simulink model "HVDC_VSC_1CPUcore_dcpl"  (Simulink 8.4)
settings: Solver=ode3  SolverMode=SingleTasking  StartTime=0.0  StopTime=70.0  FixedStep=Ts_Power  RelTol=1e-3  AbsTol=1e-2
PreLoadFcn:
  | Ts_Power=50e-6; Ts_Control=1*Ts_Power; init_cosim_IA; startup_transients_hvdc_vsc;
PostLoadFcn:
  | Ts_Power=50e-6; Ts_Control=1*Ts_Power; init_cosim_IA; startup_transients_hvdc_vsc;
InitFcn:
  | Ts_Power=50e-6; Ts_Control=1*Ts_Power; init_cosim_IA; startup_transients_hvdc_vsc;
values from neighbouring files (symbols this model uses):
  h = 5    [init_cosim_IA.m]
  intfDelay = 400.0    (= 400)    [init_cosim_IA.m]
  Ts_intf = 2*Ts_Power    [init_cosim_IA.m]
undefined symbols (not defined in the file or in its folder): CLARK, D1, Delta, dPref1_2, dPref1_2_rlimit, gcbh, level, lib_mesures, magnitude, ResistanceM, rte_drive_private_lib, rte_tsb3level_hiz_rect_cb, sps_rtmsupport, t_deblock_Pref1, t_deblock_Udref2, t_dPref1_2, t_init_AC, t_SwitchITMIdc, t_SwitchITMVdc, t_vsag_end, t_vsag_start, TSB3_hiZR
libraries: powerlib x162, powerlib_extras x71, spsVIMeasurementModel x63, rteventslib x26, op_dpl_lib x14, powerlib_meascontrol x14, rtlab x6, sps_avr x3, artemis x1
(part 9 of 11)

== system HVDC_VSC_1CPUcore_dcpl/SM_HVDC_VSC/VSC Controller (Station 1)/Discrete VSC Controller (Station 1)/Outer Active-Reactive Power and Voltage Loop/Reactive_Power_Control/AC Voltage Control Override ==
  note: Reset states when enabling
  note: AC Voltage Control Override
  note: Output is added to the regulator reference in order to maintain the AC voltage within minimum and maximum limits
  Ki_rpc_vco : Inport
  Kp_rpc_vco : Inport  Port=2
  U_max : Inport  Port=3
  U_min : Inport  Port=4
  U_meas : Inport  Port=5
  Enable : EnablePort  StatesWhenEnabling=reset
  Constant2 : Constant  Value=0.0
  Constant3 : Constant  Value=min_rpc_vco
  Constant5 : Constant
  Constant6 : Constant  Value=max_rpc_vco
  Constant7 : Constant  Value=0.0
  Constant8 : Constant
  "Int1 " : Subsystem  mask(Integrator  With  External  Dynamic  Limits (Discrete)){i_ic=0, Ts=Ts_Control}
      mask prompts: i_ic "Initial Condition:"; Ts "Sample time: (s)"
      mask Display: disp('Discrete-Time\n(Trapezoidal)\nIntegrator\n ')
  Int2 : Subsystem  mask(Integrator  With  External  Dynamic  Limits (Discrete)){i_ic=0, Ts=Ts_Control}
      mask prompts: i_ic "Initial Condition:"; Ts "Sample time: (s)"
      mask Display: disp('Discrete-Time\n(Trapezoidal)\nIntegrator\n ')
  Logical Operator : Logic  Operator=NOT  Inputs=1  AllPortsSameDT=off
  Logical Operator1 : Logic  Operator=NOT  Inputs=1  AllPortsSameDT=off
  Max=0 Min=min_rpc_vco : Saturate  UpperLimit=0  LowerLimit=min_rpc_vco
  Max=max_rpc_vco Min=0 : Saturate  UpperLimit=max_rpc_vco  LowerLimit=0
  Max=max_rpc_vco Min=min_rpc_vco : Saturate  UpperLimit=max_rpc_vco  LowerLimit=min_rpc_vco
  Product : Product  RndMeth=Zero
  Sum : Sum  Inputs=+-  SaturateOnIntegerOverflow=on
  Sum1 : Sum  Inputs=-+  SaturateOnIntegerOverflow=on
  Sum2 : Sum  Inputs=+++  SaturateOnIntegerOverflow=on
  Sum3 : Sum  SaturateOnIntegerOverflow=on
  Out : Outport
  wires:
  Product/1 -> Sum2/3
  Sum3/1 -> Product/2
  Kp_rpc_vco/1 -> Product/1
  Max=max_rpc_vco Min=0/1 -> Sum3/2
  Int2/1(Out) -> Sum2/2  "positive"
  Max=0 Min=min_rpc_vco/1 -> Sum3/1
  Logical Operator/1 -> "Int1 "/5(Hold), "Int1 "/6(Reset)
  Constant5/1 -> Logical Operator/1
  Constant2/1 -> "Int1 "/1(Max), "Int1 "/7(Reset Value)
  Constant3/1 -> "Int1 "/2(Min)
  Ki_rpc_vco/1 -> Int2/4(Ki), "Int1 "/4(Ki)
  U_max/1 -> Sum/1
  U_meas/1 -> Sum/2, Sum1/1
  Sum/1 -> Max=0 Min=min_rpc_vco/1, "Int1 "/3(In)
  Logical Operator1/1 -> Int2/5(Hold), Int2/6(Reset)
  Constant8/1 -> Logical Operator1/1
  Constant6/1 -> Int2/1(Max)
  Constant7/1 -> Int2/2(Min), Int2/7(Reset Value)
  Sum1/1 -> Max=max_rpc_vco Min=0/1, Int2/3(In)
  U_min/1 -> Sum1/2
  "Int1 "/1(Out) -> Sum2/1  "negative"
  Sum2/1 -> Max=max_rpc_vco Min=min_rpc_vco/1
  Max=max_rpc_vco Min=min_rpc_vco/1 -> Out/1

== system HVDC_VSC_1CPUcore_dcpl/SM_HVDC_VSC/VSC Controller (Station 1)/Discrete VSC Controller (Station 1)/Outer Active-Reactive Power and Voltage Loop/Reactive_Power_Control/Freeze_integrator ==
  note: Freeze Integrator
  note: Low AC voltage level
  U_meas : Inport
  Constant8 : Constant  Value=V_level_rpc
  Relational Operator : RelationalOperator  Operator=<=
  Freeze : Outport
  wires:
  U_meas/1 -> Relational Operator/1
  Relational Operator/1 -> Freeze/1
  Constant8/1 -> Relational Operator/2

== system HVDC_VSC_1CPUcore_dcpl/SM_HVDC_VSC/VSC Controller (Station 1)/Discrete VSC Controller (Station 1)/Outer Active-Reactive Power and Voltage Loop/Reactive_Power_Control/Regulator ==
  note: Regulator
  note: Reset states when enabling
  Ord : Inport
  Meas : Inport  Port=2
  Ki : Inport  Port=3
  max_out : Inport  Port=4
  min_out : Inport  Port=5
  freeze : Inport  Port=6
  Enable : EnablePort  StatesWhenEnabling=reset
  Constant1 : Constant  Value=0
  Constant2 : Constant  Value=max_i_rpc
  Constant3 : Constant  Value=min_i_rpc
  Constant5 : Constant
  Constant7 : Constant  Value=0.0
  Gain : Gain  Gain=-1  SaturateOnIntegerOverflow=on  OutDataTypeStr=Inherit: Same as input  ParamDataTypeStr=Inherit: Same as input
  Ic=0 : UnitDelay  SampleTime=Ts_Control
  Int : Subsystem  mask(Integrator  With  External  Dynamic  Limits (Discrete)){i_ic=0, Ts=Ts_Control}
      mask prompts: i_ic "Initial Condition:"; Ts "Sample time: (s)"
      mask Display: disp('Discrete-Time\n(Trapezoidal)\nIntegrator\n ')
  Kf_rpc : Constant  Value=1.0
  Logical Operator : Logic  Operator=NOT  Inputs=1  AllPortsSameDT=off
  Product2 : Product  SaturateOnIntegerOverflow=on  OutDataTypeStr=Inherit: Same as first input
  S6 : Subsystem  AncestorBlock=|  mask(Limiter with External Limits){}
      | powerlib_extras/Discrete 
      | Control Blocks/Discrete 12-Pulse
      | HVDC Control /Functions
      | (Discrete)/Current Regulator/S16/S6
      mask Display: disp('      Limiter\n')
  Sum1 : Sum  SaturateOnIntegerOverflow=on
  Sum2 : Sum  Inputs=|+-  SaturateOnIntegerOverflow=on
  Sum3 : Sum  SaturateOnIntegerOverflow=on
  Sum4 : Sum  Inputs=+-  SaturateOnIntegerOverflow=on
  Switch : Switch  Threshold=0.5  SaturateOnIntegerOverflow=on
  Out : Outport
  wires:
  Gain/1 -> Out/1
  Ic=0/1 -> Sum1/2
  Kf_rpc/1 -> Product2/1
  Logical Operator/1 -> Int/5(Hold), Int/6(Reset)
  Constant5/1 -> Logical Operator/1
  Constant1/1 -> Int/7(Reset Value)
  Constant2/1 -> Int/1(Max)
  Constant3/1 -> Int/2(Min)
  Sum1/1 -> Int/3(In)
  Ord/1 -> Sum3/1, Sum4/1
  Ki/1 -> Int/4(Ki)
  max_out/1 -> S6/1(MAX)
  min_out/1 -> S6/3(MIN)
  S6/1("  ") -> Gain/1, Sum2/1
  Sum2/1 -> Product2/2
  Product2/1 -> Ic=0/1
  Sum3/1 -> S6/2(In), Sum2/2
  Int/1(Out) -> Sum3/2
  freeze/1 -> Switch/2
  Constant7/1 -> Switch/1
  Sum4/1 -> Switch/3
  Switch/1 -> Sum1/1
  Meas/1 -> Sum4/2

== system HVDC_VSC_1CPUcore_dcpl/SM_HVDC_VSC/VSC Controller (Station 2)/Discrete VSC Controller (Station 2)/Clark Transformations/CLARK_YD/CLARK ==
  note: CLARK transformation
  abc : Inport
  Enable : EnablePort
  Fcn1 : Fcn  Expr=1/sqrt(3)*(u[2] - u[3])
  Fcn2 : Fcn  Expr=1/3*(2*u[1] - u[2] - u[3])
  Fcn3 : Fcn  Expr=1/3*(u[1] + u[2] + u[3])
  Mux : Mux  Inputs=3
  AB0 : Outport
  wires:
  Fcn2/1 -> Mux/1
  abc/1 -> Fcn1/1, Fcn3/1, Fcn2/1
  Fcn1/1 -> Mux/2
  Fcn3/1 -> Mux/3
  Mux/1 -> AB0/1

== system HVDC_VSC_1CPUcore_dcpl/SM_HVDC_VSC/VSC Controller (Station 2)/Discrete VSC Controller (Station 2)/Clark Transformations/CLARK_YD/CLARK_YD1 ==
  note: CLARK transformation - YD1
  abc : Inport
  Enable : EnablePort
  Fcn1 : Fcn  Expr=(-u[1] - u[3] + 2*u[2] )/3
  Fcn2 : Fcn  Expr=(u[1]-u[3])/sqrt(3)
  Fcn3 : Fcn  Expr=0
  Mux : Mux  Inputs=3
  AB0 : Outport
  wires:
  Fcn2/1 -> Mux/1
  abc/1 -> Fcn1/1, Fcn3/1, Fcn2/1
  Fcn1/1 -> Mux/2
  Fcn3/1 -> Mux/3
  Mux/1 -> AB0/1

== system HVDC_VSC_1CPUcore_dcpl/SM_HVDC_VSC/VSC Controller (Station 2)/Discrete VSC Controller (Station 2)/Clark Transformations/CLARK_YD/CLARK_YD11 ==
  note: CLARK transformation - YD11
  abc : Inport
  Enable : EnablePort
  Fcn1 : Fcn  Expr=(u[1] + u[2] - 2*u[3] )/3
  Fcn2 : Fcn  Expr=(u[1]-u[2])/sqrt(3)
  Fcn3 : Fcn  Expr=0
  Mux : Mux  Inputs=3
  AB0 : Outport
  wires:
  Mux/1 -> AB0/1
  Fcn3/1 -> Mux/3
  Fcn1/1 -> Mux/2
  abc/1 -> Fcn2/1, Fcn3/1, Fcn1/1
  Fcn2/1 -> Mux/1

== system HVDC_VSC_1CPUcore_dcpl/SM_HVDC_VSC/VSC Controller (Station 2)/Discrete VSC Controller (Station 2)/Clark Transformations/CLARK_YD /CLARK ==
  note: CLARK transformation
  abc : Inport
  Enable : EnablePort
  Fcn1 : Fcn  Expr=1/sqrt(3)*(u[2] - u[3])
  Fcn2 : Fcn  Expr=1/3*(2*u[1] - u[2] - u[3])
  Fcn3 : Fcn  Expr=1/3*(u[1] + u[2] + u[3])
  Mux : Mux  Inputs=3
  AB0 : Outport
  wires:
  Mux/1 -> AB0/1
  Fcn3/1 -> Mux/3
  Fcn1/1 -> Mux/2
  abc/1 -> Fcn2/1, Fcn3/1, Fcn1/1
  Fcn2/1 -> Mux/1

== system HVDC_VSC_1CPUcore_dcpl/SM_HVDC_VSC/VSC Controller (Station 2)/Discrete VSC Controller (Station 2)/Clark Transformations/CLARK_YD /CLARK_YD1 ==
  note: CLARK transformation - YD1
  abc : Inport
  Enable : EnablePort
  Fcn1 : Fcn  Expr=(-u[1] - u[3] + 2*u[2] )/3
  Fcn2 : Fcn  Expr=(u[1]-u[3])/sqrt(3)
  Fcn3 : Fcn  Expr=0
  Mux : Mux  Inputs=3
  AB0 : Outport
  wires:
  Mux/1 -> AB0/1
  Fcn3/1 -> Mux/3
  Fcn1/1 -> Mux/2
  abc/1 -> Fcn2/1, Fcn3/1, Fcn1/1
  Fcn2/1 -> Mux/1

== system HVDC_VSC_1CPUcore_dcpl/SM_HVDC_VSC/VSC Controller (Station 2)/Discrete VSC Controller (Station 2)/Clark Transformations/CLARK_YD /CLARK_YD11 ==
  note: CLARK transformation - YD11
  abc : Inport
  Enable : EnablePort
  Fcn1 : Fcn  Expr=(u[1] + u[2] - 2*u[3] )/3
  Fcn2 : Fcn  Expr=(u[1]-u[2])/sqrt(3)
  Fcn3 : Fcn  Expr=0
  Mux : Mux  Inputs=3
  AB0 : Outport
  wires:
  Fcn2/1 -> Mux/1
  abc/1 -> Fcn1/1, Fcn3/1, Fcn2/1
  Fcn1/1 -> Mux/2
  Fcn3/1 -> Mux/3
  Mux/1 -> AB0/1

== system HVDC_VSC_1CPUcore_dcpl/SM_HVDC_VSC/VSC Controller (Station 2)/Discrete VSC Controller (Station 2)/DC Voltage Balance Control/Regulator/PI_regulator  ==
  note: PI Regulator - Type 2
  note: Active Power Control
  note: max_i_apc
  note: min_i_apc
  note: Parameters
  note: Constants
  note: Ki_apc
  note: Kp_apc
  Ord : Inport
  Meas : Inport  Port=2
  Ki : Inport  Port=3
  Kp : Inport  Port=4
  Kf : Inport  Port=5
  Constant1 : Constant  Value=0
  Constant2 : Constant  Value=max_i
  Constant3 : Constant  Value=min_i
  Constant4 : Constant  Value=max_out
  Constant5 : Constant
  Constant6 : Constant  Value=min_out
  INT : Subsystem  mask(Integrator  With  External  Dynamic  Limits (Discrete)){}
      mask Display: disp('Discrete-Time\n(Trapezoidal)\nIntegrator\n ')
  Ic=0 : UnitDelay  SampleTime=Ts
  Logical Operator : Logic  Operator=NOT  Inputs=1  AllPortsSameDT=off
  Product1 : Product  SaturateOnIntegerOverflow=on  OutDataTypeStr=Inherit: Same as first input
  Product2 : Product  SaturateOnIntegerOverflow=on  OutDataTypeStr=Inherit: Same as first input
  S6 : Subsystem  AncestorBlock=|  mask(Limiter with External Limits){}
      | powerlib_extras/Discrete 
      | Control Blocks/Discrete 12-Pulse
      | HVDC Control /Functions
      | (Discrete)/Current Regulator/S16/S6
      mask Display: disp('      Limiter\n')
  Sum2 : Sum  Inputs=|+-  SaturateOnIntegerOverflow=on
  Sum3 : Sum  SaturateOnIntegerOverflow=on
  Sum4 : Sum  Inputs=+-  SaturateOnIntegerOverflow=on
  Sum5 : Sum  SaturateOnIntegerOverflow=on
  Out : Outport
  wires:
  Logical Operator/1 -> INT/6(Reset), INT/5(Hold)
  Constant5/1 -> Logical Operator/1
  Constant1/1 -> INT/7(Reset Value)
  Constant2/1 -> INT/1(Max)
  Constant3/1 -> INT/2(Min)
  Sum4/1 -> Product1/2, Sum5/1
  Meas/1 -> Sum4/2
  Ord/1 -> Sum4/1
  Ki/1 -> INT/4(Ki)
  Constant4/1 -> S6/1(MAX)
  Constant6/1 -> S6/3(MIN)
  S6/1("  ") -> Sum2/1, Out/1
  Sum2/1 -> Product2/2
  Product2/1 -> Ic=0/1
  Kf/1 -> Product2/1
  Ic=0/1 -> Sum5/2
  Sum3/1 -> S6/2(In), Sum2/2
  INT/1(Out) -> Sum3/2
  Kp/1 -> Product1/1
  Sum5/1 -> INT/3(In)
  Product1/1 -> Sum3/1

== system HVDC_VSC_1CPUcore_dcpl/SM_HVDC_VSC/VSC Controller (Station 2)/Discrete VSC Controller (Station 2)/Inner Current Loop/AC_Current_Control/PI_regulator  ==
  note: Kp_apc
  note: Ki_apc
  note: Constants
  note: Parameters
  note: min_i_apc
  note: max_i_apc
  note: Active Power Control
  note: PI Regulator - Type 2
  Ord : Inport
  Meas : Inport  Port=2
  Ki : Inport  Port=3
  Kp : Inport  Port=4
  Kf : Inport  Port=5
  Constant1 : Constant  Value=0
  Constant2 : Constant  Value=max_i
  Constant3 : Constant  Value=min_i
  Constant4 : Constant  Value=max_out
  Constant5 : Constant
  Constant6 : Constant  Value=min_out
  INT : Subsystem  mask(Integrator  With  External  Dynamic  Limits (Discrete)){}
      mask Display: disp('Discrete-Time\n(Trapezoidal)\nIntegrator\n ')
  Ic=0 : UnitDelay  SampleTime=Ts
  Logical Operator : Logic  Operator=NOT  Inputs=1  AllPortsSameDT=off
  Product1 : Product  SaturateOnIntegerOverflow=on  OutDataTypeStr=Inherit: Same as first input
  Product2 : Product  SaturateOnIntegerOverflow=on  OutDataTypeStr=Inherit: Same as first input
  S6 : Subsystem  AncestorBlock=|  mask(Limiter with External Limits){}
      | powerlib_extras/Discrete 
      | Control Blocks/Discrete 12-Pulse
      | HVDC Control /Functions
      | (Discrete)/Current Regulator/S16/S6
      mask Display: disp('      Limiter\n')
  Sum2 : Sum  Inputs=|+-  SaturateOnIntegerOverflow=on
  Sum3 : Sum  SaturateOnIntegerOverflow=on
  Sum4 : Sum  Inputs=+-  SaturateOnIntegerOverflow=on
  Sum5 : Sum  SaturateOnIntegerOverflow=on
  Out : Outport
  wires:
  Product1/1 -> Sum3/1
  Sum5/1 -> INT/3(In)
  Kp/1 -> Product1/1
  INT/1(Out) -> Sum3/2
  Sum3/1 -> Sum2/2, S6/2(In)
  Ic=0/1 -> Sum5/2
  Kf/1 -> Product2/1
  Product2/1 -> Ic=0/1
  Sum2/1 -> Product2/2
  S6/1("  ") -> Out/1, Sum2/1
  Constant6/1 -> S6/3(MIN)
  Constant4/1 -> S6/1(MAX)
  Ki/1 -> INT/4(Ki)
  Ord/1 -> Sum4/1
  Meas/1 -> Sum4/2
  Sum4/1 -> Sum5/1, Product1/2
  Constant3/1 -> INT/2(Min)
  Constant2/1 -> INT/1(Max)
  Constant1/1 -> INT/7(Reset Value)
  Constant5/1 -> Logical Operator/1
  Logical Operator/1 -> INT/5(Hold), INT/6(Reset)

== system HVDC_VSC_1CPUcore_dcpl/SM_HVDC_VSC/VSC Controller (Station 2)/Discrete VSC Controller (Station 2)/Inner Current Loop/AC_Current_Control/PI_regulator_2 ==
  note: PI Regulator - Type 2
  note: Active Power Control
  note: max_i_apc
  note: min_i_apc
  note: Parameters
  note: Constants
  note: Ki_apc
  note: Kp_apc
  Ord : Inport
  Meas : Inport  Port=2
  Ki : Inport  Port=3
  Kp : Inport  Port=4
  Kf : Inport  Port=5
  Constant1 : Constant  Value=0
  Constant2 : Constant  Value=max_i
  Constant3 : Constant  Value=min_i
  Constant4 : Constant  Value=max_out
  Constant5 : Constant
  Constant6 : Constant  Value=min_out
  INT : Subsystem  mask(Integrator  With  External  Dynamic  Limits (Discrete)){}
      mask Display: disp('Discrete-Time\n(Trapezoidal)\nIntegrator\n ')
  Ic=0 : UnitDelay  SampleTime=Ts
  Logical Operator : Logic  Operator=NOT  Inputs=1  AllPortsSameDT=off
  Product1 : Product  SaturateOnIntegerOverflow=on  OutDataTypeStr=Inherit: Same as first input
  Product2 : Product  SaturateOnIntegerOverflow=on  OutDataTypeStr=Inherit: Same as first input
  S6 : Subsystem  AncestorBlock=|  mask(Limiter with External Limits){}
      | powerlib_extras/Discrete 
      | Control Blocks/Discrete 12-Pulse
      | HVDC Control /Functions
      | (Discrete)/Current Regulator/S16/S6
      mask Display: disp('      Limiter\n')
  Sum2 : Sum  Inputs=|+-  SaturateOnIntegerOverflow=on
  Sum3 : Sum  SaturateOnIntegerOverflow=on
  Sum4 : Sum  Inputs=+-  SaturateOnIntegerOverflow=on
  Sum5 : Sum  SaturateOnIntegerOverflow=on
  Out : Outport
  wires:
  Logical Operator/1 -> INT/6(Reset), INT/5(Hold)
  Constant5/1 -> Logical Operator/1
  Constant1/1 -> INT/7(Reset Value)
  Constant2/1 -> INT/1(Max)
  Constant3/1 -> INT/2(Min)
  Sum4/1 -> Product1/2, Sum5/1
  Meas/1 -> Sum4/2
  Ord/1 -> Sum4/1
  Ki/1 -> INT/4(Ki)
  Constant4/1 -> S6/1(MAX)
  Constant6/1 -> S6/3(MIN)
  S6/1("  ") -> Sum2/1, Out/1
  Sum2/1 -> Product2/2
  Product2/1 -> Ic=0/1
  Kf/1 -> Product2/1
  Ic=0/1 -> Sum5/2
  Sum3/1 -> S6/2(In), Sum2/2
  INT/1(Out) -> Sum3/2
  Kp/1 -> Product1/1
  Sum5/1 -> INT/3(In)
  Product1/1 -> Sum3/1

== system HVDC_VSC_1CPUcore_dcpl/SM_HVDC_VSC/VSC Controller (Station 2)/Discrete VSC Controller (Station 2)/Outer Active-Reactive Power and Voltage Loop/Active_Power_Control/DC Voltage Control Override ==
  note: Output is added to the regulator reference in order to maintain the DC voltage within minimum and maximum limits
  note: DC Voltage Control Override
  note: Reset states when enabling
  Ki_apc_vco : Inport
  Kp_apc_vco : Inport  Port=2
  Udc_max : Inport  Port=3
  Udc_min : Inport  Port=4
  Udc_meas : Inport  Port=5
  Enable : EnablePort  StatesWhenEnabling=reset
  Constant2 : Constant  Value=0.0
  Constant3 : Constant  Value=min_apc_vco
  Constant5 : Constant
  Constant6 : Constant  Value=max_apc_vco
  Constant7 : Constant  Value=0.0
  Constant8 : Constant
  "Int1 " : Subsystem  mask(Integrator  With  External  Dynamic  Limits (Discrete)){i_ic=0, Ts=Ts_Control}
      mask prompts: i_ic "Initial Condition:"; Ts "Sample time: (s)"
      mask Display: disp('Discrete-Time\n(Trapezoidal)\nIntegrator\n ')
  Int2 : Subsystem  mask(Integrator  With  External  Dynamic  Limits (Discrete)){i_ic=0, Ts=Ts_Control}
      mask prompts: i_ic "Initial Condition:"; Ts "Sample time: (s)"
      mask Display: disp('Discrete-Time\n(Trapezoidal)\nIntegrator\n ')
  Logical Operator : Logic  Operator=NOT  Inputs=1  AllPortsSameDT=off
  Logical Operator1 : Logic  Operator=NOT  Inputs=1  AllPortsSameDT=off
  Max=0 Min=min_apc_vco : Saturate  UpperLimit=0  LowerLimit=min_apc_vco
  Max=max_apc_vco Min=0 : Saturate  UpperLimit=max_apc_vco  LowerLimit=0
  Max=max_apc_vco Min=min_apc_vco : Saturate  UpperLimit=max_apc_vco  LowerLimit=min_apc_vco
  Product : Product  RndMeth=Zero
  Sum : Sum  Inputs=+-  SaturateOnIntegerOverflow=on
  Sum1 : Sum  Inputs=-+  SaturateOnIntegerOverflow=on
  Sum2 : Sum  Inputs=+++  SaturateOnIntegerOverflow=on
  Sum3 : Sum  SaturateOnIntegerOverflow=on
  Out : Outport
  wires:
  Sum2/1 -> Max=max_apc_vco Min=min_apc_vco/1
  "Int1 "/1(Out) -> Sum2/1  "negative"
  Udc_min/1 -> Sum1/2
  Sum1/1 -> Int2/3(In), Max=max_apc_vco Min=0/1
  Constant7/1 -> Int2/7(Reset Value), Int2/2(Min)
  Constant6/1 -> Int2/1(Max)
  Constant8/1 -> Logical Operator1/1
  Logical Operator1/1 -> Int2/6(Reset), Int2/5(Hold)
  Sum/1 -> "Int1 "/3(In), Max=0 Min=min_apc_vco/1
  Udc_meas/1 -> Sum1/1, Sum/2
  Udc_max/1 -> Sum/1
  Ki_apc_vco/1 -> "Int1 "/4(Ki), Int2/4(Ki)
  Constant3/1 -> "Int1 "/2(Min)
  Constant2/1 -> "Int1 "/7(Reset Value), "Int1 "/1(Max)
  Constant5/1 -> Logical Operator/1
  Logical Operator/1 -> "Int1 "/6(Reset), "Int1 "/5(Hold)
  Max=0 Min=min_apc_vco/1 -> Sum3/1
  Int2/1(Out) -> Sum2/2  "positive"
  Max=max_apc_vco Min=0/1 -> Sum3/2
  Kp_apc_vco/1 -> Product/1
  Sum3/1 -> Product/2
  Product/1 -> Sum2/3
  Max=max_apc_vco Min=min_apc_vco/1 -> Out/1

== system HVDC_VSC_1CPUcore_dcpl/SM_HVDC_VSC/VSC Controller (Station 2)/Discrete VSC Controller (Station 2)/Outer Active-Reactive Power and Voltage Loop/Active_Power_Control/Freeze_integrator ==
  note: Low AC voltage level
  note: Freeze Integrator
  U_meas : Inport
  Constant8 : Constant  Value=V_level_apc
  Relational Operator : RelationalOperator  Operator=<=
  Freeze : Outport
  wires:
  Constant8/1 -> Relational Operator/2
  Relational Operator/1 -> Freeze/1
  U_meas/1 -> Relational Operator/1

== system HVDC_VSC_1CPUcore_dcpl/SM_HVDC_VSC/VSC Controller (Station 2)/Discrete VSC Controller (Station 2)/Outer Active-Reactive Power and Voltage Loop/Active_Power_Control/Ramping ==
  note: Output is reset to zero when the ramp is not enabled
  note: Ramping
  enable_ramp : Inport
  Pref : Inport  Port=2
  ramp_apc : Inport  Port=3
  Logical Operator7 : Logic  Operator=NOT  AllPortsSameDT=off
  Rate Limiter : Subsystem  AncestorBlock=my_linear/Rate Limiter (external)  mask(Rate of Change Limiter){ic=0, st=Ts_Control}
      mask prompts: ic "Initial condition (pu):"; st "Sample time (s):"
      mask help: Limit rising and falling rates of signal. When the input (R) is true the output is reset to the input (In). Rates are in p.u./s for up and -p.u./s for down.
      mask Display: disp('                Rate\n               Limiter')
  Switch : Switch  Threshold=0.5  SaturateOnIntegerOverflow=on
  zero : Constant  Value=0.0
  Pref_ramp : Outport
  wires:
  Logical Operator7/1 -> Rate Limiter/4(R)
  Switch/1 -> Rate Limiter/1(In)
  zero/1 -> Switch/3
  Pref/1 -> Switch/1
  enable_ramp/1 -> Logical Operator7/1, Switch/2
  ramp_apc/1 -> Rate Limiter/2(up_rate), Rate Limiter/3(down_rate)
  Rate Limiter/1(" ") -> Pref_ramp/1

== system HVDC_VSC_1CPUcore_dcpl/SM_HVDC_VSC/VSC Controller (Station 2)/Discrete VSC Controller (Station 2)/Outer Active-Reactive Power and Voltage Loop/Active_Power_Control/Regulator ==
  note: Regulator
  note: Reset states when enabling
  Ord : Inport
  Meas : Inport  Port=2
  Ki : Inport  Port=3
  max_out : Inport  Port=4
  min_out : Inport  Port=5
  Freeze : Inport  Port=6
  Enable : EnablePort  StatesWhenEnabling=reset
  Constant1 : Constant  Value=0
  Constant2 : Constant  Value=max_i_apc
  Constant3 : Constant  Value=min_i_apc
  Constant5 : Constant
  Constant9 : Constant  Value=0.0
  Ic=0 : UnitDelay  SampleTime=Ts_Control
  Int : Subsystem  mask(Integrator  With  External  Dynamic  Limits (Discrete)){i_ic=0, Ts=Ts_Control}
      mask prompts: i_ic "Initial Condition:"; Ts "Sample time: (s)"
      mask Display: disp('Discrete-Time\n(Trapezoidal)\nIntegrator\n ')
  Kf_apc : Constant  Value=1.0
  Logical Operator : Logic  Operator=NOT  Inputs=1  AllPortsSameDT=off
  Product2 : Product  SaturateOnIntegerOverflow=on  OutDataTypeStr=Inherit: Same as first input
  S6 : Subsystem  AncestorBlock=|  mask(Limiter with External Limits){}
      | powerlib_extras/Discrete 
      | Control Blocks/Discrete 12-Pulse
      | HVDC Control /Functions
      | (Discrete)/Current Regulator/S16/S6
      mask Display: disp('      Limiter\n')
  Sum1 : Sum  SaturateOnIntegerOverflow=on
  Sum2 : Sum  Inputs=|+-  SaturateOnIntegerOverflow=on
  Sum3 : Sum  SaturateOnIntegerOverflow=on
  Sum4 : Sum  Inputs=+-  SaturateOnIntegerOverflow=on
  Switch : Switch  Threshold=0.5  SaturateOnIntegerOverflow=on
  Out : Outport
  wires:
  Constant9/1 -> Switch/1
  Freeze/1 -> Switch/2
  Switch/1 -> Sum1/1
  Int/1(Out) -> Sum3/2
  Sum3/1 -> S6/2(In), Sum2/2
  Product2/1 -> Ic=0/1
  Sum2/1 -> Product2/2
  S6/1("  ") -> Sum2/1, Out/1
  min_out/1 -> S6/3(MIN)
  max_out/1 -> S6/1(MAX)
  Ki/1 -> Int/4(Ki)
  Sum1/1 -> Int/3(In)
  Constant3/1 -> Int/2(Min)
  Constant2/1 -> Int/1(Max)
  Constant1/1 -> Int/7(Reset Value)
  Constant5/1 -> Logical Operator/1
  Logical Operator/1 -> Int/6(Reset), Int/5(Hold)
  Kf_apc/1 -> Product2/1
  Ic=0/1 -> Sum1/2
  Ord/1 -> Sum4/1, Sum3/1
  Meas/1 -> Sum4/2
  Sum4/1 -> Switch/3

== system HVDC_VSC_1CPUcore_dcpl/SM_HVDC_VSC/VSC Controller (Station 2)/Discrete VSC Controller (Station 2)/Outer Active-Reactive Power and Voltage Loop/Current_Reference_Calculation/S1 ==
  note: Limiter
      | with external
      | limits
  MAX : Inport
  In : Inport  Port=2
  MIN : Inport  Port=3
  MinMax : MinMax  Function=max  Inputs=2  SaturateOnIntegerOverflow=on  InputSameDT=on
  MinMax1 : MinMax  Inputs=2  SaturateOnIntegerOverflow=on  InputSameDT=on
  "  " : Outport  InitialOutput=0
  wires:
  MinMax1/1 -> MinMax/2
  MAX/1 -> MinMax1/1
  MIN/1 -> MinMax/1
  MinMax/1 -> "  "/1
  In/1 -> MinMax1/2

== system HVDC_VSC_1CPUcore_dcpl/SM_HVDC_VSC/VSC Controller (Station 2)/Discrete VSC Controller (Station 2)/Outer Active-Reactive Power and Voltage Loop/Current_Reference_Calculation/S2 ==
  note: Limiter
      | with external
      | limits
  MAX : Inport
  In : Inport  Port=2
  MIN : Inport  Port=3
  MinMax : MinMax  Function=max  Inputs=2  SaturateOnIntegerOverflow=on  InputSameDT=on
  MinMax1 : MinMax  Inputs=2  SaturateOnIntegerOverflow=on  InputSameDT=on
  "  " : Outport  InitialOutput=0
  wires:
  In/1 -> MinMax1/2
  MinMax/1 -> "  "/1
  MIN/1 -> MinMax/1
  MAX/1 -> MinMax1/1
  MinMax1/1 -> MinMax/2

== system HVDC_VSC_1CPUcore_dcpl/SM_HVDC_VSC/VSC Controller (Station 2)/Discrete VSC Controller (Station 2)/Outer Active-Reactive Power and Voltage Loop/Current_Reference_Limitation/Double click here for  info ==
  note: Power System Simulation laboratory (IREQ)
  note: Current Reference Limitation
  note: The susbsytem limits the amplitude of phase current of the fundamental component to the rated current
      | of the converter.
  note: Power Control Mode
  note: DC Voltage Control Mode
  note: In power control mode, equal scaling is applied to the active and reactive power reference when a limit is imposed.
  note: In DC voltage control mode, higher priority is given to the active power when a limit is imposed.

== system HVDC_VSC_1CPUcore_dcpl/SM_HVDC_VSC/VSC Controller (Station 2)/Discrete VSC Controller (Station 2)/Outer Active-Reactive Power and Voltage Loop/DC_Voltage_Control/PI ==
  note: INTEGRATOR (Trapezoidal) with External limits & Reset & Hold
  Max : Inport
  Min : Inport  Port=2
  In : Inport  Port=3
  Ki : Inport  Port=4
  Hold : Inport  Port=5
  Reset : Inport  Port=6
  Reset Value : Inport  Port=7
  Gain : Gain  Gain=Ts* 0.5  SaturateOnIntegerOverflow=on  OutDataTypeStr=Inherit: Same as input  ParamDataTypeStr=Inherit: Same as input
  IC = 0 : UnitDelay  SampleTime=Ts
  IC = i_ic : UnitDelay  InitialCondition=i_ic  SampleTime=Ts
  Logical Operator4 : Logic  Operator=OR
  MinMax : MinMax  Inputs=2  SaturateOnIntegerOverflow=on  InputSameDT=on
  MinMax1 : MinMax  Function=max  Inputs=2  SaturateOnIntegerOverflow=on  InputSameDT=on
  Product : Product  SaturateOnIntegerOverflow=on  OutDataTypeStr=Inherit: Same as first input
  S6 : Subsystem  AncestorBlock=|  mask(Limiter with External Limits){}
      | powerlib_extras/Discrete 
      | Control Blocks/Discrete 12-Pulse
      | HVDC Control /Functions
      | (Discrete)/Current Regulator/S16/S6
      mask Display: disp('      Limiter\n')
  Sum : Sum  SaturateOnIntegerOverflow=on  InputSameDT=on  OutDataTypeStr=Inherit: Same as first input
  Sum1 : Sum  SaturateOnIntegerOverflow=on  InputSameDT=on  OutDataTypeStr=Inherit: Same as first input
  Switch2 : Switch  Threshold=0.5  SaturateOnIntegerOverflow=on  InputSameDT=on
  Switch3 : Switch  Threshold=0.5  SaturateOnIntegerOverflow=on  InputSameDT=on
  Switch7 : Switch  Threshold=0.5  SaturateOnIntegerOverflow=on  InputSameDT=on
  Out : Outport  InitialOutput=0
  wires:
  S6/1("  ") -> IC = i_ic/1, Out/1
  Gain/1 -> Product/1
  Sum1/1 -> Product/2
  Ki/1 -> Gain/1
  IC = 0/1 -> Sum1/2
  In/1 -> IC = 0/1, Sum1/1
  Product/1 -> Sum/1
  Sum/1 -> S6/2(In)
  Hold/1 -> Logical Operator4/1
  Reset/1 -> Switch7/2, Logical Operator4/2
  Logical Operator4/1 -> Switch2/2, Switch3/2
  Switch2/1 -> MinMax/1
  Max/1 -> Switch2/3, MinMax/2
  Reset Value/1 -> Switch7/1
  MinMax/1 -> S6/1(MAX)
  MinMax1/1 -> S6/3(MIN)
  Switch3/1 -> MinMax1/1
  Min/1 -> Switch3/3, MinMax1/2
  IC = i_ic/1 -> Switch7/3
  Switch7/1 -> Switch2/1, Sum/2, Switch3/1

== system HVDC_VSC_1CPUcore_dcpl/SM_HVDC_VSC/VSC Controller (Station 2)/Discrete VSC Controller (Station 2)/Outer Active-Reactive Power and Voltage Loop/DC_Voltage_Control/S6 ==
  note: Limiter
      | with external
      | limits
  MAX : Inport
  In : Inport  Port=2
  MIN : Inport  Port=3
  MinMax : MinMax  Function=max  Inputs=2  SaturateOnIntegerOverflow=on  InputSameDT=on
  MinMax1 : MinMax  Inputs=2  SaturateOnIntegerOverflow=on  InputSameDT=on
  "  " : Outport  InitialOutput=0
  wires:
  MinMax1/1 -> MinMax/2
  MAX/1 -> MinMax1/1
  MIN/1 -> MinMax/1
  MinMax/1 -> "  "/1
  In/1 -> MinMax1/2

== system HVDC_VSC_1CPUcore_dcpl/SM_HVDC_VSC/VSC Controller (Station 2)/Discrete VSC Controller (Station 2)/Outer Active-Reactive Power and Voltage Loop/Reactive_Power_Control/AC Voltage Control Override ==
  note: Reset states when enabling
  note: AC Voltage Control Override
  note: Output is added to the regulator reference in order to maintain the AC voltage within minimum and maximum limits
  Ki_rpc_vco : Inport
  Kp_rpc_vco : Inport  Port=2
  U_max : Inport  Port=3
  U_min : Inport  Port=4
  U_meas : Inport  Port=5
  Enable : EnablePort  StatesWhenEnabling=reset
  Constant2 : Constant  Value=0.0
  Constant3 : Constant  Value=min_rpc_vco
  Constant5 : Constant
  Constant6 : Constant  Value=max_rpc_vco
  Constant7 : Constant  Value=0.0
  Constant8 : Constant
  "Int1 " : Subsystem  mask(Integrator  With  External  Dynamic  Limits (Discrete)){i_ic=0, Ts=Ts_Control}
      mask prompts: i_ic "Initial Condition:"; Ts "Sample time: (s)"
      mask Display: disp('Discrete-Time\n(Trapezoidal)\nIntegrator\n ')
  Int2 : Subsystem  mask(Integrator  With  External  Dynamic  Limits (Discrete)){i_ic=0, Ts=Ts_Control}
      mask prompts: i_ic "Initial Condition:"; Ts "Sample time: (s)"
      mask Display: disp('Discrete-Time\n(Trapezoidal)\nIntegrator\n ')
  Logical Operator : Logic  Operator=NOT  Inputs=1  AllPortsSameDT=off
  Logical Operator1 : Logic  Operator=NOT  Inputs=1  AllPortsSameDT=off
  Max=0 Min=min_rpc_vco : Saturate  UpperLimit=0  LowerLimit=min_rpc_vco
  Max=max_rpc_vco Min=0 : Saturate  UpperLimit=max_rpc_vco  LowerLimit=0
  Max=max_rpc_vco Min=min_rpc_vco : Saturate  UpperLimit=max_rpc_vco  LowerLimit=min_rpc_vco
  Product : Product  RndMeth=Zero
  Sum : Sum  Inputs=+-  SaturateOnIntegerOverflow=on
  Sum1 : Sum  Inputs=-+  SaturateOnIntegerOverflow=on
  Sum2 : Sum  Inputs=+++  SaturateOnIntegerOverflow=on
  Sum3 : Sum  SaturateOnIntegerOverflow=on
  Out : Outport
  wires:
  Product/1 -> Sum2/3
  Sum3/1 -> Product/2
  Kp_rpc_vco/1 -> Product/1
  Max=max_rpc_vco Min=0/1 -> Sum3/2
  Int2/1(Out) -> Sum2/2  "positive"
  Max=0 Min=min_rpc_vco/1 -> Sum3/1
  Logical Operator/1 -> "Int1 "/5(Hold), "Int1 "/6(Reset)
  Constant5/1 -> Logical Operator/1
  Constant2/1 -> "Int1 "/1(Max), "Int1 "/7(Reset Value)
  Constant3/1 -> "Int1 "/2(Min)
  Ki_rpc_vco/1 -> Int2/4(Ki), "Int1 "/4(Ki)
  U_max/1 -> Sum/1
  U_meas/1 -> Sum/2, Sum1/1
  Sum/1 -> Max=0 Min=min_rpc_vco/1, "Int1 "/3(In)
  Logical Operator1/1 -> Int2/5(Hold), Int2/6(Reset)
  Constant8/1 -> Logical Operator1/1
  Constant6/1 -> Int2/1(Max)
  Constant7/1 -> Int2/2(Min), Int2/7(Reset Value)
  Sum1/1 -> Max=max_rpc_vco Min=0/1, Int2/3(In)
  U_min/1 -> Sum1/2
  "Int1 "/1(Out) -> Sum2/1  "negative"
  Sum2/1 -> Max=max_rpc_vco Min=min_rpc_vco/1
  Max=max_rpc_vco Min=min_rpc_vco/1 -> Out/1

== system HVDC_VSC_1CPUcore_dcpl/SM_HVDC_VSC/VSC Controller (Station 2)/Discrete VSC Controller (Station 2)/Outer Active-Reactive Power and Voltage Loop/Reactive_Power_Control/Freeze_integrator ==
  note: Freeze Integrator
  note: Low AC voltage level
  U_meas : Inport
  Constant8 : Constant  Value=V_level_rpc
  Relational Operator : RelationalOperator  Operator=<=
  Freeze : Outport
  wires:
  U_meas/1 -> Relational Operator/1
  Relational Operator/1 -> Freeze/1
  Constant8/1 -> Relational Operator/2

== system HVDC_VSC_1CPUcore_dcpl/SM_HVDC_VSC/VSC Controller (Station 2)/Discrete VSC Controller (Station 2)/Outer Active-Reactive Power and Voltage Loop/Reactive_Power_Control/Regulator ==
  note: Regulator
  note: Reset states when enabling
  Ord : Inport
  Meas : Inport  Port=2
  Ki : Inport  Port=3
  max_out : Inport  Port=4
  min_out : Inport  Port=5
  freeze : Inport  Port=6
  Enable : EnablePort  StatesWhenEnabling=reset
  Constant1 : Constant  Value=0
  Constant2 : Constant  Value=max_i_rpc
  Constant3 : Constant  Value=min_i_rpc
  Constant5 : Constant
  Constant7 : Constant  Value=0.0
  Gain : Gain  Gain=-1  SaturateOnIntegerOverflow=on  OutDataTypeStr=Inherit: Same as input  ParamDataTypeStr=Inherit: Same as input
  Ic=0 : UnitDelay  SampleTime=Ts_Control
  Int : Subsystem  mask(Integrator  With  External  Dynamic  Limits (Discrete)){i_ic=0, Ts=Ts_Control}
      mask prompts: i_ic "Initial Condition:"; Ts "Sample time: (s)"
      mask Display: disp('Discrete-Time\n(Trapezoidal)\nIntegrator\n ')
  Kf_rpc : Constant  Value=1.0
  Logical Operator : Logic  Operator=NOT  Inputs=1  AllPortsSameDT=off
  Product2 : Product  SaturateOnIntegerOverflow=on  OutDataTypeStr=Inherit: Same as first input
  S6 : Subsystem  AncestorBlock=|  mask(Limiter with External Limits){}
      | powerlib_extras/Discrete 
      | Control Blocks/Discrete 12-Pulse
      | HVDC Control /Functions
      | (Discrete)/Current Regulator/S16/S6
      mask Display: disp('      Limiter\n')
  Sum1 : Sum  SaturateOnIntegerOverflow=on
  Sum2 : Sum  Inputs=|+-  SaturateOnIntegerOverflow=on
  Sum3 : Sum  SaturateOnIntegerOverflow=on
  Sum4 : Sum  Inputs=+-  SaturateOnIntegerOverflow=on
  Switch : Switch  Threshold=0.5  SaturateOnIntegerOverflow=on
  Out : Outport
  wires:
  Gain/1 -> Out/1
  Ic=0/1 -> Sum1/2
  Kf_rpc/1 -> Product2/1
  Logical Operator/1 -> Int/5(Hold), Int/6(Reset)
  Constant5/1 -> Logical Operator/1
  Constant1/1 -> Int/7(Reset Value)
  Constant2/1 -> Int/1(Max)
  Constant3/1 -> Int/2(Min)
  Sum1/1 -> Int/3(In)
  Ord/1 -> Sum3/1, Sum4/1
  Ki/1 -> Int/4(Ki)
  max_out/1 -> S6/1(MAX)
  min_out/1 -> S6/3(MIN)
  S6/1("  ") -> Gain/1, Sum2/1
  Sum2/1 -> Product2/2
  Product2/1 -> Ic=0/1
  Sum3/1 -> S6/2(In), Sum2/2
  Int/1(Out) -> Sum3/2
  freeze/1 -> Switch/2
  Constant7/1 -> Switch/1
  Sum4/1 -> Switch/3
  Switch/1 -> Sum1/1
  Meas/1 -> Sum4/2

== system HVDC_VSC_1CPUcore_dcpl/SM_HVDC_VSC/VSC Controller (Station 1)/Discrete VSC Controller (Station 1)/DC Voltage Balance Control/Regulator/PI_regulator /INT ==
  note: INTEGRATOR (Trapezoidal) with External limits & Reset & Hold
  Max : Inport
  Min : Inport  Port=2
  In : Inport  Port=3
  Ki : Inport  Port=4
  Hold : Inport  Port=5
  Reset : Inport  Port=6
  Reset Value : Inport  Port=7
  Gain : Gain  Gain=Ts* 0.5  SaturateOnIntegerOverflow=on  OutDataTypeStr=Inherit: Same as input  ParamDataTypeStr=Inherit: Same as input
  IC = 0 : UnitDelay  SampleTime=Ts
  IC = i_ic : UnitDelay  InitialCondition=i_ic  SampleTime=Ts
  Logical Operator4 : Logic  Operator=OR
  MinMax : MinMax  Inputs=2  SaturateOnIntegerOverflow=on  InputSameDT=on
  MinMax1 : MinMax  Function=max  Inputs=2  SaturateOnIntegerOverflow=on  InputSameDT=on
  Product : Product  SaturateOnIntegerOverflow=on  OutDataTypeStr=Inherit: Same as first input
  S6 : Subsystem  AncestorBlock=|  mask(Limiter with External Limits){}
      | powerlib_extras/Discrete 
      | Control Blocks/Discrete 12-Pulse
      | HVDC Control /Functions
      | (Discrete)/Current Regulator/S16/S6
      mask Display: disp('      Limiter\n')
  Sum : Sum  SaturateOnIntegerOverflow=on  InputSameDT=on  OutDataTypeStr=Inherit: Same as first input
  Sum1 : Sum  SaturateOnIntegerOverflow=on  InputSameDT=on  OutDataTypeStr=Inherit: Same as first input
  Switch2 : Switch  Threshold=0.5  SaturateOnIntegerOverflow=on  InputSameDT=on
  Switch3 : Switch  Threshold=0.5  SaturateOnIntegerOverflow=on  InputSameDT=on
  Switch7 : Switch  Threshold=0.5  SaturateOnIntegerOverflow=on  InputSameDT=on
  Out : Outport  InitialOutput=0
  wires:
  Switch7/1 -> Switch3/1, Sum/2, Switch2/1
  IC = i_ic/1 -> Switch7/3
  Min/1 -> MinMax1/2, Switch3/3
  Switch3/1 -> MinMax1/1
  MinMax1/1 -> S6/3(MIN)
  MinMax/1 -> S6/1(MAX)
  Reset Value/1 -> Switch7/1
  Max/1 -> MinMax/2, Switch2/3
  Switch2/1 -> MinMax/1
  Logical Operator4/1 -> Switch3/2, Switch2/2
  Reset/1 -> Logical Operator4/2, Switch7/2
  Hold/1 -> Logical Operator4/1
  Sum/1 -> S6/2(In)
  Product/1 -> Sum/1
  In/1 -> Sum1/1, IC = 0/1
  IC = 0/1 -> Sum1/2
  Ki/1 -> Gain/1
  Sum1/1 -> Product/2
  Gain/1 -> Product/1
  S6/1("  ") -> Out/1, IC = i_ic/1

== system HVDC_VSC_1CPUcore_dcpl/SM_HVDC_VSC/VSC Controller (Station 1)/Discrete VSC Controller (Station 1)/DC Voltage Balance Control/Regulator/PI_regulator /S6 ==
  note: Limiter
      | with external
      | limits
  MAX : Inport
  In : Inport  Port=2
  MIN : Inport  Port=3
  MinMax : MinMax  Function=max  Inputs=2  SaturateOnIntegerOverflow=on  InputSameDT=on
  MinMax1 : MinMax  Inputs=2  SaturateOnIntegerOverflow=on  InputSameDT=on
  "  " : Outport  InitialOutput=0
  wires:
  In/1 -> MinMax1/2
  MinMax/1 -> "  "/1
  MIN/1 -> MinMax/1
  MAX/1 -> MinMax1/1
  MinMax1/1 -> MinMax/2

== system HVDC_VSC_1CPUcore_dcpl/SM_HVDC_VSC/VSC Controller (Station 1)/Discrete VSC Controller (Station 1)/Inner Current Loop/AC_Current_Control/PI_regulator /INT ==
  note: INTEGRATOR (Trapezoidal) with External limits & Reset & Hold
  Max : Inport
  Min : Inport  Port=2
  In : Inport  Port=3
  Ki : Inport  Port=4
  Hold : Inport  Port=5
  Reset : Inport  Port=6
  Reset Value : Inport  Port=7
  Gain : Gain  Gain=Ts* 0.5  SaturateOnIntegerOverflow=on  OutDataTypeStr=Inherit: Same as input  ParamDataTypeStr=Inherit: Same as input
  IC = 0 : UnitDelay  SampleTime=Ts
  IC = i_ic : UnitDelay  InitialCondition=i_ic  SampleTime=Ts
  Logical Operator4 : Logic  Operator=OR
  MinMax : MinMax  Inputs=2  SaturateOnIntegerOverflow=on  InputSameDT=on
  MinMax1 : MinMax  Function=max  Inputs=2  SaturateOnIntegerOverflow=on  InputSameDT=on
  Product : Product  SaturateOnIntegerOverflow=on  OutDataTypeStr=Inherit: Same as first input
  S6 : Subsystem  AncestorBlock=|  mask(Limiter with External Limits){}
      | powerlib_extras/Discrete 
      | Control Blocks/Discrete 12-Pulse
      | HVDC Control /Functions
      | (Discrete)/Current Regulator/S16/S6
      mask Display: disp('      Limiter\n')
  Sum : Sum  SaturateOnIntegerOverflow=on  InputSameDT=on  OutDataTypeStr=Inherit: Same as first input
  Sum1 : Sum  SaturateOnIntegerOverflow=on  InputSameDT=on  OutDataTypeStr=Inherit: Same as first input
  Switch2 : Switch  Threshold=0.5  SaturateOnIntegerOverflow=on  InputSameDT=on
  Switch3 : Switch  Threshold=0.5  SaturateOnIntegerOverflow=on  InputSameDT=on
  Switch7 : Switch  Threshold=0.5  SaturateOnIntegerOverflow=on  InputSameDT=on
  Out : Outport  InitialOutput=0
  wires:
  S6/1("  ") -> IC = i_ic/1, Out/1
  Gain/1 -> Product/1
  Sum1/1 -> Product/2
  Ki/1 -> Gain/1
  IC = 0/1 -> Sum1/2
  In/1 -> IC = 0/1, Sum1/1
  Product/1 -> Sum/1
  Sum/1 -> S6/2(In)
  Hold/1 -> Logical Operator4/1
  Reset/1 -> Switch7/2, Logical Operator4/2
  Logical Operator4/1 -> Switch2/2, Switch3/2
  Switch2/1 -> MinMax/1
  Max/1 -> Switch2/3, MinMax/2
  Reset Value/1 -> Switch7/1
  MinMax/1 -> S6/1(MAX)
  MinMax1/1 -> S6/3(MIN)
  Switch3/1 -> MinMax1/1
  Min/1 -> Switch3/3, MinMax1/2
  IC = i_ic/1 -> Switch7/3
  Switch7/1 -> Switch2/1, Sum/2, Switch3/1

== system HVDC_VSC_1CPUcore_dcpl/SM_HVDC_VSC/VSC Controller (Station 1)/Discrete VSC Controller (Station 1)/Inner Current Loop/AC_Current_Control/PI_regulator /S6 ==
  note: Limiter
      | with external
      | limits
  MAX : Inport
  In : Inport  Port=2
  MIN : Inport  Port=3
  MinMax : MinMax  Function=max  Inputs=2  SaturateOnIntegerOverflow=on  InputSameDT=on
  MinMax1 : MinMax  Inputs=2  SaturateOnIntegerOverflow=on  InputSameDT=on
  "  " : Outport  InitialOutput=0
  wires:
  MinMax1/1 -> MinMax/2
  MAX/1 -> MinMax1/1
  MIN/1 -> MinMax/1
  MinMax/1 -> "  "/1
  In/1 -> MinMax1/2

== system HVDC_VSC_1CPUcore_dcpl/SM_HVDC_VSC/VSC Controller (Station 1)/Discrete VSC Controller (Station 1)/Inner Current Loop/AC_Current_Control/PI_regulator_2/INT ==
  note: INTEGRATOR (Trapezoidal) with External limits & Reset & Hold
  Max : Inport
  Min : Inport  Port=2
  In : Inport  Port=3
  Ki : Inport  Port=4
  Hold : Inport  Port=5
  Reset : Inport  Port=6
  Reset Value : Inport  Port=7
  Gain : Gain  Gain=Ts* 0.5  SaturateOnIntegerOverflow=on  OutDataTypeStr=Inherit: Same as input  ParamDataTypeStr=Inherit: Same as input
  IC = 0 : UnitDelay  SampleTime=Ts
  IC = i_ic : UnitDelay  InitialCondition=i_ic  SampleTime=Ts
  Logical Operator4 : Logic  Operator=OR
  MinMax : MinMax  Inputs=2  SaturateOnIntegerOverflow=on  InputSameDT=on
  MinMax1 : MinMax  Function=max  Inputs=2  SaturateOnIntegerOverflow=on  InputSameDT=on
  Product : Product  SaturateOnIntegerOverflow=on  OutDataTypeStr=Inherit: Same as first input
  S6 : Subsystem  AncestorBlock=|  mask(Limiter with External Limits){}
      | powerlib_extras/Discrete 
      | Control Blocks/Discrete 12-Pulse
      | HVDC Control /Functions
      | (Discrete)/Current Regulator/S16/S6
      mask Display: disp('      Limiter\n')
  Sum : Sum  SaturateOnIntegerOverflow=on  InputSameDT=on  OutDataTypeStr=Inherit: Same as first input
  Sum1 : Sum  SaturateOnIntegerOverflow=on  InputSameDT=on  OutDataTypeStr=Inherit: Same as first input
  Switch2 : Switch  Threshold=0.5  SaturateOnIntegerOverflow=on  InputSameDT=on
  Switch3 : Switch  Threshold=0.5  SaturateOnIntegerOverflow=on  InputSameDT=on
  Switch7 : Switch  Threshold=0.5  SaturateOnIntegerOverflow=on  InputSameDT=on
  Out : Outport  InitialOutput=0
  wires:
  Switch7/1 -> Switch3/1, Sum/2, Switch2/1
  IC = i_ic/1 -> Switch7/3
  Min/1 -> MinMax1/2, Switch3/3
  Switch3/1 -> MinMax1/1
  MinMax1/1 -> S6/3(MIN)
  MinMax/1 -> S6/1(MAX)
  Reset Value/1 -> Switch7/1
  Max/1 -> MinMax/2, Switch2/3
  Switch2/1 -> MinMax/1
  Logical Operator4/1 -> Switch3/2, Switch2/2
  Reset/1 -> Logical Operator4/2, Switch7/2
  Hold/1 -> Logical Operator4/1
  Sum/1 -> S6/2(In)
  Product/1 -> Sum/1
  In/1 -> Sum1/1, IC = 0/1
  IC = 0/1 -> Sum1/2
  Ki/1 -> Gain/1
  Sum1/1 -> Product/2
  Gain/1 -> Product/1
  S6/1("  ") -> Out/1, IC = i_ic/1

== system HVDC_VSC_1CPUcore_dcpl/SM_HVDC_VSC/VSC Controller (Station 1)/Discrete VSC Controller (Station 1)/Inner Current Loop/AC_Current_Control/PI_regulator_2/S6 ==
  note: Limiter
      | with external
      | limits
  MAX : Inport
  In : Inport  Port=2
  MIN : Inport  Port=3
  MinMax : MinMax  Function=max  Inputs=2  SaturateOnIntegerOverflow=on  InputSameDT=on
  MinMax1 : MinMax  Inputs=2  SaturateOnIntegerOverflow=on  InputSameDT=on
  "  " : Outport  InitialOutput=0
  wires:
  In/1 -> MinMax1/2
  MinMax/1 -> "  "/1
  MIN/1 -> MinMax/1
  MAX/1 -> MinMax1/1
  MinMax1/1 -> MinMax/2

== system HVDC_VSC_1CPUcore_dcpl/SM_HVDC_VSC/VSC Controller (Station 1)/Discrete VSC Controller (Station 1)/Outer Active-Reactive Power and Voltage Loop/Active_Power_Control/DC Voltage Control Override/Int1  ==
  note: INTEGRATOR (Trapezoidal) with External limits & Reset & Hold
  Max : Inport
  Min : Inport  Port=2
  In : Inport  Port=3
  Ki : Inport  Port=4
  Hold : Inport  Port=5
  Reset : Inport  Port=6
  Reset Value : Inport  Port=7
  Gain : Gain  Gain=Ts* 0.5  SaturateOnIntegerOverflow=on  OutDataTypeStr=Inherit: Same as input  ParamDataTypeStr=Inherit: Same as input
  IC = 0 : UnitDelay  SampleTime=Ts
  IC = i_ic : UnitDelay  InitialCondition=i_ic  SampleTime=Ts
  Logical Operator4 : Logic  Operator=OR
  MinMax : MinMax  Inputs=2  SaturateOnIntegerOverflow=on  InputSameDT=on
  MinMax1 : MinMax  Function=max  Inputs=2  SaturateOnIntegerOverflow=on  InputSameDT=on
  Product : Product  SaturateOnIntegerOverflow=on  OutDataTypeStr=Inherit: Same as first input
  S6 : Subsystem  AncestorBlock=|  mask(Limiter with External Limits){}
      | powerlib_extras/Discrete 
      | Control Blocks/Discrete 12-Pulse
      | HVDC Control /Functions
      | (Discrete)/Current Regulator/S16/S6
      mask Display: disp('      Limiter\n')
  Sum : Sum  SaturateOnIntegerOverflow=on  InputSameDT=on  OutDataTypeStr=Inherit: Same as first input
  Sum1 : Sum  SaturateOnIntegerOverflow=on  InputSameDT=on  OutDataTypeStr=Inherit: Same as first input
  Switch2 : Switch  Threshold=0.5  SaturateOnIntegerOverflow=on  InputSameDT=on
  Switch3 : Switch  Threshold=0.5  SaturateOnIntegerOverflow=on  InputSameDT=on
  Switch7 : Switch  Threshold=0.5  SaturateOnIntegerOverflow=on  InputSameDT=on
  Out : Outport  InitialOutput=0
  wires:
  Switch7/1 -> Switch3/1, Sum/2, Switch2/1
  IC = i_ic/1 -> Switch7/3
  Min/1 -> MinMax1/2, Switch3/3
  Switch3/1 -> MinMax1/1
  MinMax1/1 -> S6/3(MIN)
  MinMax/1 -> S6/1(MAX)
  Reset Value/1 -> Switch7/1
  Max/1 -> MinMax/2, Switch2/3
  Switch2/1 -> MinMax/1
  Logical Operator4/1 -> Switch3/2, Switch2/2
  Reset/1 -> Logical Operator4/2, Switch7/2
  Hold/1 -> Logical Operator4/1
  Sum/1 -> S6/2(In)
  Product/1 -> Sum/1
  In/1 -> Sum1/1, IC = 0/1
  IC = 0/1 -> Sum1/2
  Ki/1 -> Gain/1
  Sum1/1 -> Product/2
  Gain/1 -> Product/1
  S6/1("  ") -> Out/1, IC = i_ic/1

== system HVDC_VSC_1CPUcore_dcpl/SM_HVDC_VSC/VSC Controller (Station 1)/Discrete VSC Controller (Station 1)/Outer Active-Reactive Power and Voltage Loop/Active_Power_Control/DC Voltage Control Override/Int2 ==
  note: INTEGRATOR (Trapezoidal) with External limits & Reset & Hold
  Max : Inport
  Min : Inport  Port=2
  In : Inport  Port=3
  Ki : Inport  Port=4
  Hold : Inport  Port=5
  Reset : Inport  Port=6
  Reset Value : Inport  Port=7
  Gain : Gain  Gain=Ts* 0.5  SaturateOnIntegerOverflow=on  OutDataTypeStr=Inherit: Same as input  ParamDataTypeStr=Inherit: Same as input
  IC = 0 : UnitDelay  SampleTime=Ts
  IC = i_ic : UnitDelay  InitialCondition=i_ic  SampleTime=Ts
  Logical Operator4 : Logic  Operator=OR
  MinMax : MinMax  Inputs=2  SaturateOnIntegerOverflow=on  InputSameDT=on
  MinMax1 : MinMax  Function=max  Inputs=2  SaturateOnIntegerOverflow=on  InputSameDT=on
  Product : Product  SaturateOnIntegerOverflow=on  OutDataTypeStr=Inherit: Same as first input
  S6 : Subsystem  AncestorBlock=|  mask(Limiter with External Limits){}
      | powerlib_extras/Discrete 
      | Control Blocks/Discrete 12-Pulse
      | HVDC Control /Functions
      | (Discrete)/Current Regulator/S16/S6
      mask Display: disp('      Limiter\n')
  Sum : Sum  SaturateOnIntegerOverflow=on  InputSameDT=on  OutDataTypeStr=Inherit: Same as first input
  Sum1 : Sum  SaturateOnIntegerOverflow=on  InputSameDT=on  OutDataTypeStr=Inherit: Same as first input
  Switch2 : Switch  Threshold=0.5  SaturateOnIntegerOverflow=on  InputSameDT=on
  Switch3 : Switch  Threshold=0.5  SaturateOnIntegerOverflow=on  InputSameDT=on
  Switch7 : Switch  Threshold=0.5  SaturateOnIntegerOverflow=on  InputSameDT=on
  Out : Outport  InitialOutput=0
  wires:
  S6/1("  ") -> IC = i_ic/1, Out/1
  Gain/1 -> Product/1
  Sum1/1 -> Product/2
  Ki/1 -> Gain/1
  IC = 0/1 -> Sum1/2
  In/1 -> IC = 0/1, Sum1/1
  Product/1 -> Sum/1
  Sum/1 -> S6/2(In)
  Hold/1 -> Logical Operator4/1
  Reset/1 -> Switch7/2, Logical Operator4/2
  Logical Operator4/1 -> Switch2/2, Switch3/2
  Switch2/1 -> MinMax/1
  Max/1 -> Switch2/3, MinMax/2
  Reset Value/1 -> Switch7/1
  MinMax/1 -> S6/1(MAX)
  MinMax1/1 -> S6/3(MIN)
  Switch3/1 -> MinMax1/1
  Min/1 -> Switch3/3, MinMax1/2
  IC = i_ic/1 -> Switch7/3
  Switch7/1 -> Switch2/1, Sum/2, Switch3/1

== system HVDC_VSC_1CPUcore_dcpl/SM_HVDC_VSC/VSC Controller (Station 1)/Discrete VSC Controller (Station 1)/Outer Active-Reactive Power and Voltage Loop/Active_Power_Control/Ramping/Rate Limiter ==
  note: Silvano Casoria
      | Laboratoire simulation de reseaux, IREQ
  note: Max= 4
      | Min =1
  note: IC=ic
  note: Rate Limiter with external rates
  In : Inport
  up_rate : Inport  Port=2
  down_rate : Inport  Port=3
  R : Inport  Port=4
  Abs : Abs  SaturateOnIntegerOverflow=on
  Constant3 : Constant
  Data Type Conversion1 : DataTypeConversion  SaturateOnIntegerOverflow=on  RndMeth=Zero
  Data Type Conversion2 : DataTypeConversion  SaturateOnIntegerOverflow=on  RndMeth=Zero
  Data Type Conversion3 : DataTypeConversion  SaturateOnIntegerOverflow=on  RndMeth=Zero
  Gain1 : Gain  Gain=2  SaturateOnIntegerOverflow=on  OutDataTypeStr=Inherit: Same as input  ParamDataTypeStr=Inherit: Same as input
  Gain2 : Gain  Gain=3  SaturateOnIntegerOverflow=on  OutDataTypeStr=Inherit: Same as input  ParamDataTypeStr=Inherit: Same as input
  Gain3 : Gain  Gain=st  SaturateOnIntegerOverflow=on  OutDataTypeStr=Inherit: Same as input  ParamDataTypeStr=Inherit: Same as input
  Gain4 : Gain  Gain=-st  SaturateOnIntegerOverflow=on  OutDataTypeStr=Inherit: Same as input  ParamDataTypeStr=Inherit: Same as input
  Multiport Switch : MultiPortSwitch  Inputs=4  SaturateOnIntegerOverflow=on  InputSameDT=on
  Relational Operator : RelationalOperator  Operator=>  InputSameDT=on
  Relational Operator2 : RelationalOperator  Operator=<  InputSameDT=on
  Saturation : Saturate  UpperLimit=4  LowerLimit=1
  Sum : Sum  Inputs=+-  SaturateOnIntegerOverflow=on  InputSameDT=on  OutDataTypeStr=Inherit: Same as first input
  Sum1 : Sum  Inputs=++++  SaturateOnIntegerOverflow=on  InputSameDT=on  OutDataTypeStr=Inherit: Same as first input
  Sum2 : Sum  SaturateOnIntegerOverflow=on  InputSameDT=on  OutDataTypeStr=Inherit: Same as first input
  Sum3 : Sum  SaturateOnIntegerOverflow=on  InputSameDT=on  OutDataTypeStr=Inherit: Same as first input
  Unit Delay : UnitDelay  InitialCondition=ic  SampleTime=st
  " " : Outport  InitialOutput=0
  wires:
  Data Type Conversion3/1 -> Gain2/1
  Data Type Conversion2/1 -> Sum1/1
  Data Type Conversion1/1 -> Gain1/1
  Abs/1 -> Gain4/1
  down_rate/1 -> Abs/1
  up_rate/1 -> Gain3/1
  Unit Delay/1 -> Sum/2, Sum2/1, Sum3/1
  Gain3/1 -> Relational Operator/2, Sum2/2
  Gain4/1 -> Relational Operator2/2, Sum3/2
  Multiport Switch/1 -> Unit Delay/1, " "/1
  Sum/1 -> Relational Operator/1, Relational Operator2/1  "Rate"
  Relational Operator2/1 -> Data Type Conversion1/1
  In/1 -> Sum/1, Multiport Switch/2, Multiport Switch/5
  Sum2/1 -> Multiport Switch/3
  Sum3/1 -> Multiport Switch/4
  R/1 -> Data Type Conversion3/1
  Sum1/1 -> Saturation/1
  Saturation/1 -> Multiport Switch/1
  Gain1/1 -> Sum1/2
  Relational Operator/1 -> Data Type Conversion2/1
  Constant3/1 -> Sum1/4
  Gain2/1 -> Sum1/3
